simulink model "punto"  (R2020a)
settings: Solver=VariableStepAuto  StartTime=0.0  StopTime=20  RelTol=1e-3
settings Model: Creator=sht  LastModifiedBy=sht

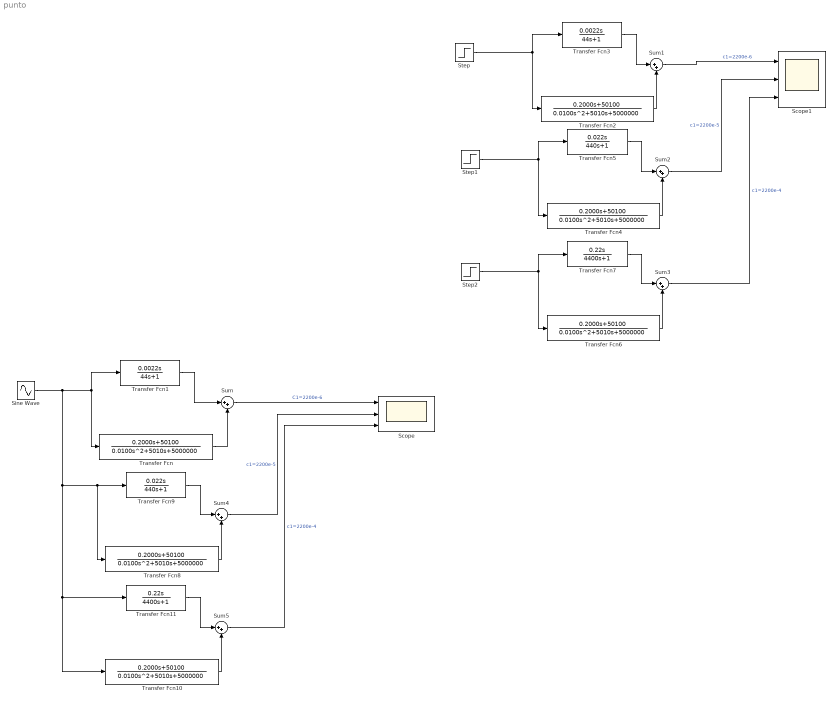
== system punto ==
  Scope : Scope  NumInputPorts=3
  Scope1 : Scope  NumInputPorts=3
  Sine Wave : Sin  Amplitude=120  Frequency=60  SampleTime=0.1
  Step : Step  After=20  SampleTime=0.01
  Step1 : Step  After=20  SampleTime=0.01
  Step2 : Step  After=20  SampleTime=0.01
  Sum{,1..5} (6 alike) : Sum  Inputs=|++
  Transfer Fcn{,2,4,6,8,10} (6 alike) : TransferFcn  Numerator=|  Denominator=[0.0100 5010 5000000]
      | [0.2000
      | 50100]
  Transfer Fcn1 : TransferFcn  Numerator=[0.0022 0]  Denominator=[44 1]
  Transfer Fcn11 : TransferFcn  Numerator=[0.22 0]  Denominator=[4400 1]
  Transfer Fcn3 : TransferFcn  Numerator=[0.0022 0]  Denominator=[44 1]
  Transfer Fcn5 : TransferFcn  Numerator=[0.022 0]  Denominator=[440 1]
  Transfer Fcn7 : TransferFcn  Numerator=[0.22 0]  Denominator=[4400 1]
  Transfer Fcn9 : TransferFcn  Numerator=[0.022 0]  Denominator=[440 1]
  wires:
  Transfer Fcn/1 -> Sum/2
  Transfer Fcn1/1 -> Sum/1
  Sum/1 -> Scope/1  "C1=2200e-6"
  Sum1/1 -> Scope1/1  "c1=2200e-6"
  Transfer Fcn2/1 -> Sum1/2
  Transfer Fcn3/1 -> Sum1/1
  Step/1 -> Transfer Fcn3/1, Transfer Fcn2/1
  Transfer Fcn4/1 -> Sum2/2
  Sum2/1 -> Scope1/2  "c1=2200e-5"
  Transfer Fcn5/1 -> Sum2/1
  Step1/1 -> Transfer Fcn5/1, Transfer Fcn4/1
  Transfer Fcn6/1 -> Sum3/2
  Transfer Fcn7/1 -> Sum3/1
  Step2/1 -> Transfer Fcn7/1, Transfer Fcn6/1
  Sum3/1 -> Scope1/3  "c1=2200e-4"
  Transfer Fcn9/1 -> Sum4/1
  Sum4/1 -> Scope/2  "c1=2200e-5"
  Transfer Fcn8/1 -> Sum4/2
  Transfer Fcn10/1 -> Sum5/2
  Sum5/1 -> Scope/3  "c1=2200e-4"
  Transfer Fcn11/1 -> Sum5/1
  Sine Wave/1 -> Transfer Fcn1/1, Transfer Fcn/1, Transfer Fcn11/1, Transfer Fcn10/1, Transfer Fcn8/1, Transfer Fcn9/1
